simulink model "stepper_sim"  (Simulink 7.1)
settings: Solver=FixedStepDiscrete  StartTime=0.0  StopTime=240  FixedStep=0.1  RelTol=1e-3
libraries: arduino_io_lib x3, simulink x3
settings Model: Creator=gcampa  LastModifiedBy=gcampa
settings OptimizationCC: InitFltsAndDblsToZero=off
settings DebuggingCC: StrictBusMsg=ErrorLevel1
settings GRTTargetCC: CPPClassGenCompliant=off

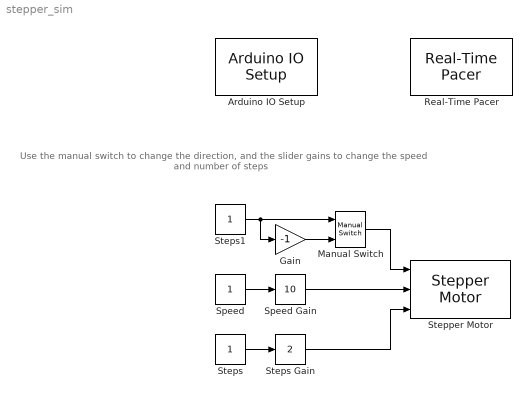
== system stepper_sim ==
  note: Use the manual switch to change the direction,
      | and the slider gains to change the speed and number of steps
  Arduino IO Setup : arduino_io_lib/Arduino IO Setup  Priority=3  arduinoVar=Arduino1  comPort=COM9
  Gain : Gain  Gain=-1
  Manual Switch : simulink/Signal Routing/Manual Switch  SystemSampleTime=-1  sw=0  action=0  varsize=off
  Real-Time Pacer : arduino_io_lib/Real-Time Pacer  simTimePerRealTime=1
  Speed : Constant
  Speed Gain : simulink/Math Operations/Slider Gain  SystemSampleTime=-1  low=0  gain=10  high=60
  Stepper Motor : arduino_io_lib/Stepper Motor  arduinoVar=Arduino1  motorNum=1  motionStyle=single  sendOnChange=on  T=0.1
  Steps : Constant
  Steps Gain : simulink/Math Operations/Slider Gain  SystemSampleTime=-1  low=0  gain=2  high=10
  Steps1 : Constant
  wires:
  Steps/1 -> Steps Gain/1
  Speed/1 -> Speed Gain/1
  Manual Switch/1 -> Stepper Motor/1
  Steps1/1 -> Manual Switch/1, Gain/1
  Gain/1 -> Manual Switch/2
  Steps Gain/1 -> Stepper Motor/3
  Speed Gain/1 -> Stepper Motor/2
